simulink model "DiagramadebloquesLTI"  (R2019a)
settings: Solver=VariableStepAuto  StartTime=0.0  StopTime=10.0  RelTol=1e-3
values from neighbouring files (symbols this model uses):
  beq = (bm+bl/r^2)    [Calculo.m]    (also in Untitled4.m; funciontrans.m)
  Jeq = (Jm+Jl/r^2)    [Calculo.m]    (also in Untitled4.m)
  lambda_m_r = 0.01546    [Datos.m]
  Ld = 6.6e-3    (= 0.0066)    [Datos.m]
  Lq = 5.8e-3    (= 0.0058)    [Datos.m]
  Pp = 3    [Datos.m]
  r = 314.3008    [Datos.m]
  Rs = Rsref*(1+alfa_cu*(Ts-40))    [Calculo.m]    (also in Datos.m = 1.05978; Untitled4.m = 1.02)
settings Model: Creator=renzo  LastModifiedBy=renzo

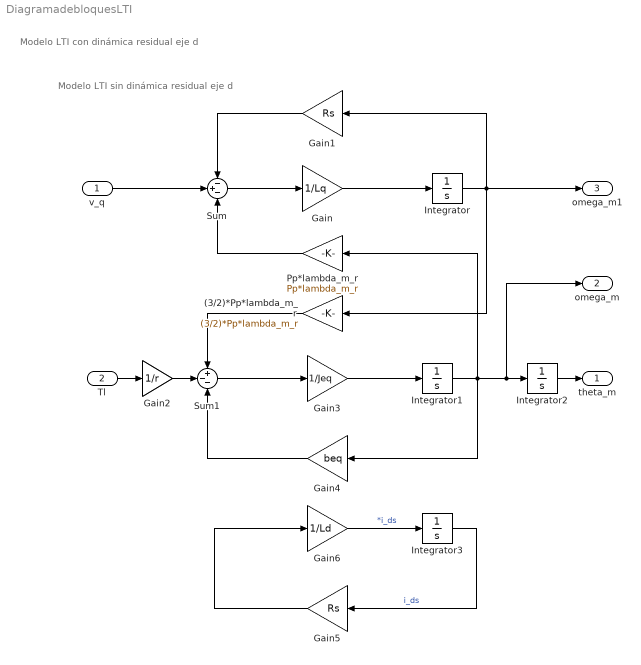
== system DiagramadebloquesLTI ==
  note: Modelo LTI con dinámica residual eje d
  note: Modelo LTI sin dinámica residual eje d
  v_q : Inport
  Tl : Inport  Port=2
  (3/2)*Pp*lambda_m_r : Gain  Gain=(3/2)*Pp*lambda_m_r
  Gain : Gain  Gain=1/Lq
  Gain1 : Gain  Gain=Rs
  Gain2 : Gain  Gain=1/r
  Gain3 : Gain  Gain=1/Jeq
  Gain4 : Gain  Gain=beq
  Gain5 : Gain  Gain=Rs
  Gain6 : Gain  Gain=1/Ld
  Integrator{,1..3} (4 alike) : Integrator
  Pp*lambda_m_r : Gain  Gain=Pp*lambda_m_r
  Sum : Sum  Inputs=-+-
  Sum1 : Sum  Inputs=+--
  theta_m : Outport
  omega_m : Outport  Port=2
  omega_m1 : Outport  Port=3
  wires:
  v_q/1 -> Sum/2
  Sum/1 -> Gain/1
  Gain/1 -> Integrator/1
  Integrator/1 -> omega_m1/1, (3/2)*Pp*lambda_m_r/1, Gain1/1
  Gain1/1 -> Sum/1
  Tl/1 -> Gain2/1
  Gain2/1 -> Sum1/2
  Sum1/1 -> Gain3/1
  Gain3/1 -> Integrator1/1
  Integrator1/1 -> omega_m/1, Integrator2/1, Pp*lambda_m_r/1, Gain4/1
  Gain4/1 -> Sum1/3
  (3/2)*Pp*lambda_m_r/1 -> Sum1/1
  Pp*lambda_m_r/1 -> Sum/3
  Integrator2/1 -> theta_m/1
  Integrator3/1 -> Gain5/1  "i_ds"
  Gain5/1 -> Gain6/1
  Gain6/1 -> Integrator3/1  "*i_ds"
